simulink model "ex10impsliding"  (R2025b)
settings: Solver=ode4  StartTime=0.0  StopTime=10.0  FixedStep=0.05  RelTol=1e-3
values from neighbouring files (symbols this model uses):
  x0 = [-7/2;4]    [ex10.m]    (also in ex12.m = [rp;vp]; ex13.m = [rp;vp]; ex5.m = [1.7524, 2.8131, 2.1589])
settings Model: Creator=Esteban  LastModifiedBy=Esteban

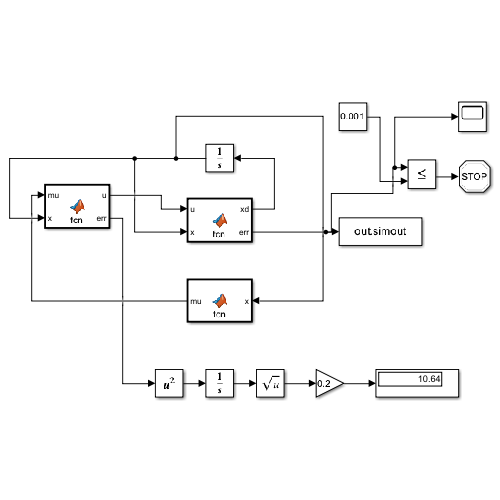
[thumbnail: Simulink's stored preview of the top-level diagram]
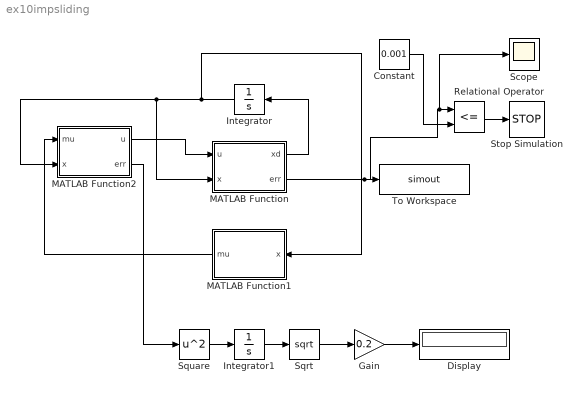
== system ex10impsliding ==
  Constant : Constant  Value=0.001
  Display : Display
  Gain : Gain  Gain=0.2
  Integrator : Integrator  InitialCondition=x0
  Integrator1 : Integrator
  MATLAB Function : MATLAB Function  TreatAsAtomicUnit=on
  MATLAB Function1 : MATLAB Function  TreatAsAtomicUnit=on
  MATLAB Function2 : MATLAB Function  TreatAsAtomicUnit=on
  Relational Operator : RelationalOperator  Operator=<=  OutDataTypeStr=boolean  RndMeth=Simplest  InputSameDT=off
  Scope : Scope
      settings: ActiveDisplayYMinimum=-0.15875036539267431  ActiveDisplayYMaximum=0.71546029118646248
  Sqrt : Sqrt
  Square : Math  Operator=square
  Stop Simulation : Stop
  To Workspace : ToWorkspace  VariableName=simout  SaveFormat=Timeseries  SampleTime=-1
  wires:
  MATLAB Function/1(xd) -> Integrator/1
  Integrator/1 -> MATLAB Function1/1(x), MATLAB Function/2(x), MATLAB Function2/2(x)
  MATLAB Function1/1(mu) -> MATLAB Function2/1(mu)
  MATLAB Function/2(err) -> Scope/1, Relational Operator/1, To Workspace/1
  MATLAB Function2/1(u) -> MATLAB Function/1(u)
  MATLAB Function2/2(err) -> Square/1
  Square/1 -> Integrator1/1
  Integrator1/1 -> Sqrt/1
  Sqrt/1 -> Gain/1
  Constant/1 -> Relational Operator/2
  Relational Operator/1 -> Stop Simulation/1
  Gain/1 -> Display/1

== matlab function ex10impsliding/MATLAB Function1 ==
  data: x input; mu output
function mu = fcn(x)

mu = [x(1);x(2)];

== matlab function ex10impsliding/MATLAB Function ==
  data: xd output; u input; err output; x input
function [xd,err] = fcn(u,x)

xd = [x(2);
    0.2*x(1)^3+x(1)-u-3*x(2)];

y=x(1);

err = norm(y);

== matlab function ex10impsliding/MATLAB Function2 ==
  data: mu input; u output; x input; err output
function [u,err]  = fcn(mu,x)

k1 = 5;
k2 = 12;
n = 1;

s = mu(2)+k2*mu(1);

v = -k2*mu(2) - k1*tanh(s*n);

u = x(1)^3/5 + x(1) - v - 3*x(2);

err = norm(u);
